simulink library "Springs_Axle2_Linear"  (R2026a)
settings: Solver=VariableStepAuto
undefined symbols (not defined in the file): Spring
libraries: fl_lib x4, Spring_Basics x4
Description:
  | Component of Simscape Vehicle Templates Library
  | 
  | Copyright 2018-2026 The MathWorks, Inc.
settings Model: Creator=smiller  LastModifiedBy=smiller

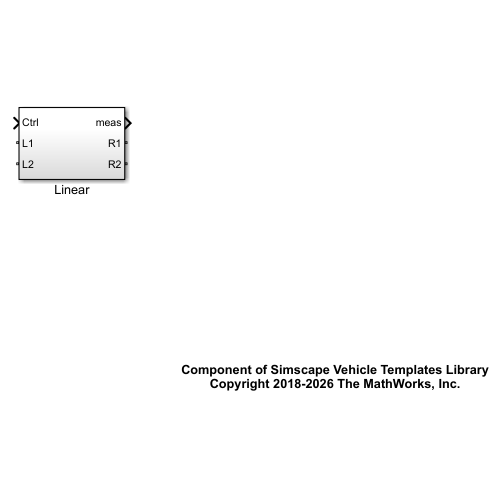
[thumbnail: Simulink's stored preview of the top-level diagram]
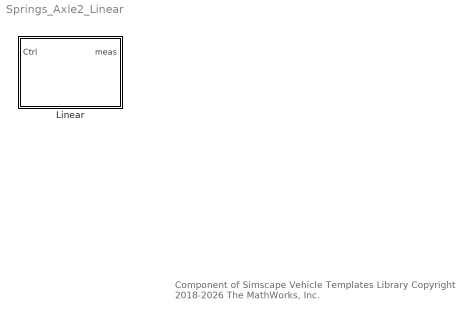
== system Springs_Axle2_Linear ==
  note: Component of Simscape Vehicle Templates Library
      | Copyright 2018-2026 The MathWorks, Inc.
  Linear : Subsystem  VariantControl=Linear

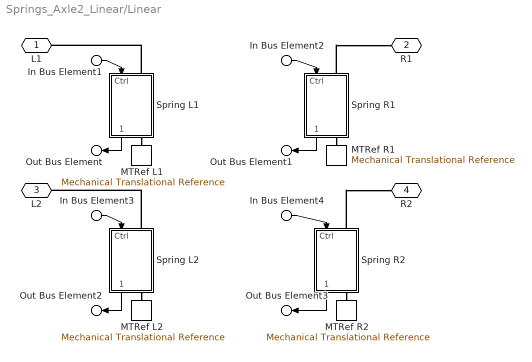
== system Springs_Axle2_Linear/Linear ==
  In Bus Element1 : Inport  PortName=Ctrl  Element=L1
  In Bus Element2 : Inport  PortName=Ctrl  Element=R1
  In Bus Element3 : Inport  PortName=Ctrl  Element=L2
  In Bus Element4 : Inport  PortName=Ctrl  Element=R2
  MTRef L1 : fl_lib/Mechanical/Translational Elements/Mechanical Translational Reference
  MTRef L2 : fl_lib/Mechanical/Translational Elements/Mechanical Translational Reference
  MTRef R1 : fl_lib/Mechanical/Translational Elements/Mechanical Translational Reference
  MTRef R2 : fl_lib/Mechanical/Translational Elements/Mechanical Translational Reference
  Spring L1 : Subsystem  mask{Spring=Spring.Axle1}
      mask prompts: Spring "Spring Parameters"
  Spring L2 : Subsystem  mask{Spring=Spring.Axle2}
      mask prompts: Spring "Spring Parameters"
  Spring R1 : Subsystem  mask{Spring=Spring.Axle1}
      mask prompts: Spring "Spring Parameters"
  Spring R2 : Subsystem  mask{Spring=Spring.Axle2}
      mask prompts: Spring "Spring Parameters"
  L1 : PMIOPort  Side=Left
  R1 : PMIOPort  Port=2  Side=Right
  L2 : PMIOPort  Port=3  Side=Left
  R2 : PMIOPort  Port=4  Side=Right
  Out Bus Element : Outport  VectorParamsAs1DForOutWhenUnconnected=off  PortName=meas  Element=L1
  Out Bus Element1 : Outport  VectorParamsAs1DForOutWhenUnconnected=off  PortName=meas  Element=R1
  Out Bus Element2 : Outport  VectorParamsAs1DForOutWhenUnconnected=off  PortName=meas  Element=L2
  Out Bus Element3 : Outport  VectorParamsAs1DForOutWhenUnconnected=off  PortName=meas  Element=R2
  wires:
  In Bus Element1/1 -> Spring L1/1(Ctrl)
  Spring L1/1(meas) -> Out Bus Element/1
  In Bus Element2/1 -> Spring R1/1(Ctrl)
  Spring R1/1(meas) -> Out Bus Element1/1
  In Bus Element3/1 -> Spring L2/1(Ctrl)
  Spring L2/1(meas) -> Out Bus Element2/1
  In Bus Element4/1 -> Spring R2/1(Ctrl)
  Spring R2/1(meas) -> Out Bus Element3/1
  connections:
  Spring R1/LConn1 -- R1/RConn1
  Spring R1/RConn1 -- MTRef R1/LConn1
  Spring R2/LConn1 -- R2/RConn1
  Spring R2/RConn1 -- MTRef R2/LConn1
  Spring L2/LConn1 -- L2/RConn1
  Spring L2/RConn1 -- MTRef L2/LConn1
  Spring L1/LConn1 -- L1/RConn1
  Spring L1/RConn1 -- MTRef L1/LConn1

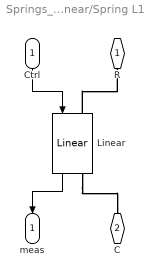
== system Springs_Axle2_Linear/Linear/Spring L1 ==
  Ctrl : Inport
  Linear : Spring_Basics/Linear  VariantControl=Linear  spr_def0=Spring.xPreload.Value  spr_k=Spring.K.Value  spr_hp_top=Spring.sTop.Value  spr_hp_bot=Spring.sBottom.Value
  R : PMIOPort  Side=Left
  C : PMIOPort  Port=2  Side=Right
  meas : Outport  VectorParamsAs1DForOutWhenUnconnected=off
  wires:
  Linear/1 -> meas/1
  Ctrl/1 -> Linear/1
  connections:
  Linear/LConn1 -- R/RConn1
  Linear/RConn1 -- C/RConn1

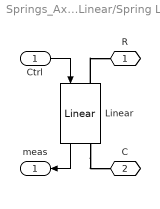
== system Springs_Axle2_Linear/Linear/Spring L2 ==
  Ctrl : Inport
  Linear : Spring_Basics/Linear  VariantControl=Linear  spr_def0=Spring.xPreload.Value  spr_k=Spring.K.Value  spr_hp_top=Spring.sTop.Value  spr_hp_bot=Spring.sBottom.Value
  R : PMIOPort  Side=Left
  C : PMIOPort  Port=2  Side=Right
  meas : Outport  VectorParamsAs1DForOutWhenUnconnected=off
  wires:
  Ctrl/1 -> Linear/1
  Linear/1 -> meas/1
  connections:
  Linear/RConn1 -- C/RConn1
  Linear/LConn1 -- R/RConn1

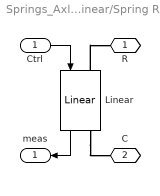
== system Springs_Axle2_Linear/Linear/Spring R1 ==
  Ctrl : Inport
  Linear : Spring_Basics/Linear  VariantControl=Linear  spr_def0=Spring.xPreload.Value  spr_k=Spring.K.Value  spr_hp_top=Spring.sTop.Value  spr_hp_bot=Spring.sBottom.Value
  R : PMIOPort  Side=Left
  C : PMIOPort  Port=2  Side=Right
  meas : Outport  VectorParamsAs1DForOutWhenUnconnected=off
  wires:
  Ctrl/1 -> Linear/1
  Linear/1 -> meas/1
  connections:
  Linear/RConn1 -- C/RConn1
  Linear/LConn1 -- R/RConn1

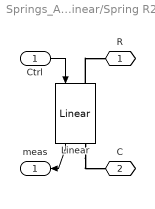
== system Springs_Axle2_Linear/Linear/Spring R2 ==
  Ctrl : Inport
  Linear : Spring_Basics/Linear  VariantControl=Linear  spr_def0=Spring.xPreload.Value  spr_k=Spring.K.Value  spr_hp_top=Spring.sTop.Value  spr_hp_bot=Spring.sBottom.Value
  R : PMIOPort  Side=Left
  C : PMIOPort  Port=2  Side=Right
  meas : Outport  VectorParamsAs1DForOutWhenUnconnected=off
  wires:
  Linear/1 -> meas/1
  Ctrl/1 -> Linear/1
  connections:
  Linear/LConn1 -- R/RConn1
  Linear/RConn1 -- C/RConn1
